simulink model "BE_EGAL_04"  (R2024b)
settings: Solver=ode45  StartTime=0.0  StopTime=1000  RelTol=1e-3  EnableMultiTasking=on
values from neighbouring files (symbols this model uses):
  Constellation = exp(1i*pi*(1+2*kc)/4)    [init_ISI.m]
undefined symbols (not defined in the file or in its folder): dfilt, Kegal, NCoeffs, Tfinal
libraries: dspobslib x3, commdigbbndam3 x3, commsink2 x2, commchan3 x1, dspstat3 x1, dspswit3 x1, commrandsrc3 x1
settings Model: Creator=Epsilon_2  LastModifiedBy=paulj
settings SolverCC: AlgebraicLoopSolver=TrustRegion
settings DataIOCC: LimitDataPoints=on  SaveFormat=Array  SignalLoggingSaveFormat=ModelDataLogs  SaveOutput=off  SaveTime=off  ReturnWorkspaceOutputs=off  SignalLoggingName=sigsOut
settings OptimizationCC: ExpressionDepthLimit=2147483647  InitFltsAndDblsToZero=on  LifeSpan=inf
settings DebuggingCC: SaveWithParameterizedLinksMsg=none  UnderspecifiedInitializationDetection=Classic  MergeDetectMultiDrivingBlocksExec=none  SignalResolutionControl=TryResolveAllWithWarning  MultiTaskDSMMsg=warning  MultiTaskCondExecSysMsg=none  FcnCallInpInsideContextMsg=warning  UnconnectedInputMsg=warning  UnconnectedOutputMsg=warning  UnconnectedLineMsg=warning  StateNameClashWarn=warning  SFUnexpectedBacktrackingDiag=warning  SFNoUnconditionalDefaultTransitionDiag=warning  SFExecutionAtInitializationDiag=none  ArithmeticOperatorsInVariantConditions=warning
settings HardwareCC: ProdBitPerPointer=32  ProdBitPerSizeT=32  ProdBitPerPtrDiffT=32  ProdLargestAtomicFloat=None  ProdIntDivRoundTo=Undefined  ProdEndianess=Unspecified  ProdWordSize=32  ProdHWDeviceType=32-bit Generic  TargetUnknown=on
settings ModelReferenceCC: PropagateSignalLabelsOutOfModel=off
settings RTWCC: GPUComputeCapability=3.5
settings CodeAppCC: StateflowObjectComments=on
settings GRTTargetCC: TargetFcnLib=ansi_tfl_tmw.mat  TargetLangStandard=C89/C90 (ANSI)  ModelReferenceCompliant=off  CombineOutputUpdateFcns=off  MatFileLogging=off  GRTInterface=on
settings ConfigComp: CovMetricSettings=dw  CovSaveCumulativeToWorkspaceVar=on  CovSaveSingleToWorkspaceVar=on

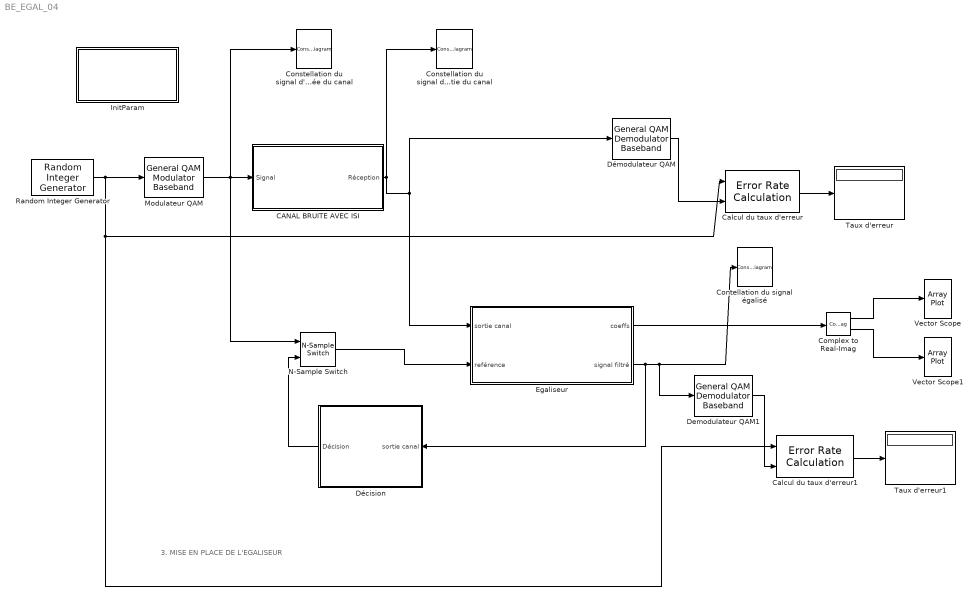
== system BE_EGAL_04 ==
  note: 3. MISE EN PLACE DE L'EGALISEUR
  CANAL BRUITE AVEC ISI : Subsystem
  Calcul du taux d'erreur : commsink2/Error Rate Calculation  N=0  st_delay=0  cp_mode=Entire frame  subframe=[]  PMode=Port  WsName=ErrorVec  RsMode2=off  stop=off  numErr=100  maxBits=1e6
  Calcul du taux d'erreur1 : commsink2/Error Rate Calculation  N=0  st_delay=0  cp_mode=Entire frame  subframe=[]  PMode=Port  WsName=ErrorVec  RsMode2=off  stop=off  numErr=100  maxBits=1e6
  Complex to Real-Imag : ComplexToRealImag
  Constellation du signal d'entrée du canal : ConstellationDiagram  Tag=ScatterPlot  WindowPosition=[382.000000,84.000000,600.000000,600.000000,]  Visible=on  ScopeFrameLocation=window  SymbolsToDisplaySource=Property  SymbolsToDisplay=1000  XLimits=[-1.47,1.47]  YLimits=[-1.38,1.38]  FigPos=[232 118 560 560]
  Constellation du signal de sortie du canal : ConstellationDiagram  Tag=ScatterPlot  WindowPosition=[463.000000,136.000000,600.000000,600.000000,]  Visible=on  ScopeFrameLocation=window  SymbolsToDisplaySource=Property  SymbolsToDisplay=1000  XLimits=[-1.47,1.47]  YLimits=[-1.38,1.38]  FigPos=[232 118 560 560]
  Contellation du signal égalisé : ConstellationDiagram  Tag=ScatterPlot  WindowPosition=[1161.000000,252.000000,600.000000,600.000000,]  Visible=on  ScopeFrameLocation=window  SymbolsToDisplaySource=Property  SymbolsToDisplay=1000  XLimits=[-1.47,1.47]  YLimits=[-1.38,1.38]  FigPos=[232 118 560 560]
  Demodulateur QAM1 : commdigbbndam3/General QAM Demodulator Baseband  SigCon=Constellation  OutType=Integer  DecType=Hard decision  VarSource=Dialog  Variance=1  outDtypeBit=Inherit via internal rule  outDtype=double  roundingMode=Floor  overflowMode=Wrap  OvFlMode=off  OvFlModeLastStrValue=off  sigConstWordLen=16  sigConstDataTypeStr=Inherit: Same word length as input  sigConstLastDataTypeStr=Inherit: Same word length as input  accum1WordLen=32  accum1FracLen=30  prodInWordLen=32  prodInFracLen=30  prodInDataTypeStr=Inherit: Same as accumulator 1  prodInLastDataTypeStr=Inherit: Same as accumulator 1  prodOutWordLen=32  prodOutFracLen=30  accum2WordLen=32  accum2FracLen=30  accum3WordLen=32  accum3FracLen=30  nsiWordLen=32  nsiFracLen=30  nsiDataTypeStr=Inherit: Same as accumulator 3  nsiLastDataTypeStr=Inherit: Same as accumulator 3  invn0WordLen=16  invn0FracLen=8  invn0DataTypeStr=Inherit: Same word length as input  invn0LastDataTypeStr=Inherit: Same word length as input  outputWordLen=32  outputFracLen=30
  Décision : Subsystem
  "Démodulateur QAM " : commdigbbndam3/General QAM Demodulator Baseband  SigCon=Constellation  OutType=Integer  DecType=Hard decision  VarSource=Dialog  Variance=1  outDtypeBit=Inherit via internal rule  outDtype=double  roundingMode=Floor  overflowMode=Wrap  OvFlMode=off  OvFlModeLastStrValue=off  sigConstWordLen=16  sigConstDataTypeStr=Inherit: Same word length as input  sigConstLastDataTypeStr=Inherit: Same word length as input  accum1WordLen=32  accum1FracLen=30  prodInWordLen=32  prodInFracLen=30  prodInDataTypeStr=Inherit: Same as accumulator 1  prodInLastDataTypeStr=Inherit: Same as accumulator 1  prodOutWordLen=32  prodOutFracLen=30  accum2WordLen=32  accum2FracLen=30  accum3WordLen=32  accum3FracLen=30  nsiWordLen=32  nsiFracLen=30  nsiDataTypeStr=Inherit: Same as accumulator 3  nsiLastDataTypeStr=Inherit: Same as accumulator 3  invn0WordLen=16  invn0FracLen=8  invn0DataTypeStr=Inherit: Same word length as input  invn0LastDataTypeStr=Inherit: Same word length as input  outputWordLen=32  outputFracLen=30
  Egaliseur : Subsystem
  InitParam : Subsystem  mask{Tech=1, Tfinal=1000, Mconst=4, NumCanal=[1 0.75 0.56 0.42 0.32 0.24 0.18], SNRcanal=100, NCoeffs=9, Kegal=0.04}
      mask prompts: Tech "Période de symbole"; Tfinal "Temps de simulation"; Mconst "Taille de la constellation de la modulation QAM : M (2^k)"; NumCanal "Modele RIF du canal"; SNRcanal "SNR du canal (en dB)"; NCoeffs "Nb de coefficients de l'égalisateur"; Kegal "Gain de l'égalisateur"
      mask help: Use the following mask to select the different parameters for the simulation.
      mask init:
      | eStr = init_ISI(gcb);
      mask Display: disp('Initialisation')
  "Modulateur QAM " : commdigbbndam3/General QAM Modulator Baseband  SigCon=Constellation  outDtype=double  outWordLen=16  outUDDataType=sfix(16)  outFracLenMode=Best precision  outFracLen=15  outDataTypeStr=double  outLastDataTypeStr=double
  N-Sample Switch : dspswit3/N-Sample Switch  N=Tfinal/10  reset=off  TriggerType=Rising edge  Ts=-1
  Random Integer Generator : commrandsrc3/Random Integer Generator  SetSize=4  SeedSource=Auto  Seed=0  SampleTime=1  SamplesPerFrame=1  OutputDataType=double  SimulateUsing=Interpreted execution
  Taux d'erreur : Display
  Taux d'erreur1 : Display
  Vector Scope : ArrayPlot  WindowPosition=[108.000000,461.000000,531.000000,480.000000,]  Visible=on  ScopeFrameLocation=window  PlotType=Line  XLabel=Time  YLimits=[-0.9705 1.2189]
  Vector Scope1 : ArrayPlot  WindowPosition=[688.000000,480.000000,484.000000,479.000000,]  Visible=on  ScopeFrameLocation=window  PlotType=Line  XLabel=Time  YLimits=[-0.0041 0.004]
  wires:
  CANAL BRUITE AVEC ISI/1(Réception) -> Constellation du signal de sortie du canal/1, "Démodulateur QAM "/1, Egaliseur/1(sortie canal)
  Random Integer Generator/1 -> "Modulateur QAM "/1, Calcul du taux d'erreur/1, Calcul du taux d'erreur1/1
  "Modulateur QAM "/1 -> N-Sample Switch/1, CANAL BRUITE AVEC ISI/1(Signal), Constellation du signal d'entrée du canal/1
  Calcul du taux d'erreur/1 -> Taux d'erreur/1
  "Démodulateur QAM "/1 -> Calcul du taux d'erreur/2
  Egaliseur/1(coeffs) -> Complex to Real-Imag/1
  Complex to Real-Imag/1 -> Vector Scope/1
  Complex to Real-Imag/2 -> Vector Scope1/1
  Calcul du taux d'erreur1/1 -> Taux d'erreur1/1
  Demodulateur QAM1/1 -> Calcul du taux d'erreur1/2
  Egaliseur/2(signal filtré) -> Décision/1(sortie canal), Demodulateur QAM1/1, Contellation du signal égalisé/1
  Décision/1(Décision) -> N-Sample Switch/2
  N-Sample Switch/1 -> Egaliseur/2(reférence)

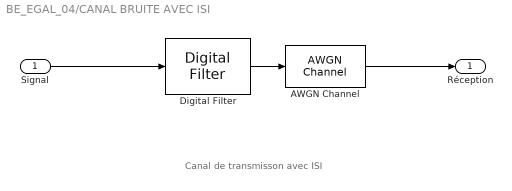
== system BE_EGAL_04/CANAL BRUITE AVEC ISI ==
  note: Canal de transmisson avec ISI
  Signal : Inport
  AWGN Channel : commchan3/AWGN Channel  LegacyMode=on  NoiseMethod="Signal to noise ratio  (SNR)"  noiseMode="Signal to noise ratio  (SNR)"  EbNo=10  EsNo=10  SNR=SNRcanal  BitsPerSymbol=1  SignalPower=1  SamplesPerSymbol=1  SymbolPeriod=1  VarianceSource=Parameter  Variance=1  RandomStream=Global stream  Seed=67  SimulateUsing=Code generation
  Digital Filter : dspobslib/Digital Filter  TypePopup=FIR (all zeros)  IIRFiltStruct=Direct form II transposed  AllPoleFiltStruct=Direct form  FIRFiltStruct=Direct form  CoeffSource=Specify via dialog  NumCoeffs=NumCanal  DenCoeffs=[1 0.1]  BiQuadCoeffs=[1 0.3 0.4 1 0.1 0.2]  LatticeCoeffs=[0.2 0.4]  denIgnore=on  FiltPerSampPopup=One filter per sample  IC=0  ICnum=0  ICden=0  roundingMode=Floor  overflowMode=off  ScaleValues=1  scaleValueFracLength=14  stageInFracLength=15  stageOutFracLength=15  FilterSource=Specify via dialog  dfiltObjectName=dfilt.dffir([1 2 1])  InputProcessing=Columns as channels (frame based)
  Réception : Outport
  wires:
  Digital Filter/1 -> AWGN Channel/1
  AWGN Channel/1 -> Réception/1
  Signal/1 -> Digital Filter/1

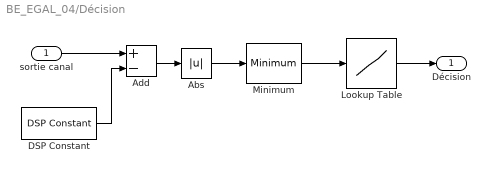
== system BE_EGAL_04/Décision ==
  sortie canal : Inport
  Abs : Abs  SaturateOnIntegerOverflow=off
  Add : Sum  Inputs=+-
  DSP Constant : dspobslib/DSP Constant  Value=Constellation  SampleMode=Discrete  discreteOutput=Sample-based (interpret vectors as 1-D)  continuousOutput=Sample-based  sampTime=inf  framePeriod=2  dataType=Inherit from 'Constant value'  isSigned=on  wordLen=16  udDataType=sfix(16)  fracBitsMode=Best precision  numFracBits=15  InterpretAs1D=-inf  Ts=-inf  FramebasedOutput=-inf
  Lookup Table : Lookup  InputValues=[1:4]  Table=Constellation  LookUpMeth=Use Input Nearest  SaturateOnIntegerOverflow=off
  Minimum : dspstat3/Minimum  operation=minimum  fcn=Index  indexBase=One  operateOver=Each column  Dimension=1  InputProcessing=Columns as channels (frame based)  reset=None  roiEnable=off  roiType=Rectangles  roiPortion=Entire ROI  roiOutput=Individual statistics for each ROI  roiFlag=off  roundingMode=Floor  overflowMode=off
  Décision : Outport
  wires:
  Minimum/1 -> Lookup Table/1
  Lookup Table/1 -> Décision/1
  Abs/1 -> Minimum/1
  Add/1 -> Abs/1
  DSP Constant/1 -> Add/2
  sortie canal/1 -> Add/1

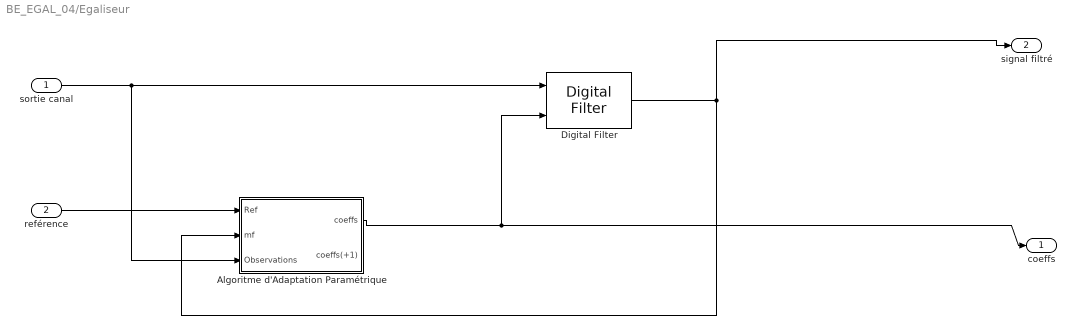
== system BE_EGAL_04/Egaliseur ==
  sortie canal : Inport
  reférence : Inport  Port=2
  Algoritme d'Adaptation Paramétrique : Subsystem
  Digital Filter : dspobslib/Digital Filter  TypePopup=FIR (all zeros)  IIRFiltStruct=Direct form II transposed  AllPoleFiltStruct=Direct form  FIRFiltStruct=Direct form  CoeffSource=Input port(s)  NumCoeffs=1  DenCoeffs=[1 0.1]  BiQuadCoeffs=[1 0.3 0.4 1 0.1 0.2]  LatticeCoeffs=[0.2 0.4]  denIgnore=on  FiltPerSampPopup=One filter per sample  IC=0  ICnum=0  ICden=0  roundingMode=Floor  overflowMode=off  ScaleValues=1  scaleValueFracLength=14  stageInFracLength=15  stageOutFracLength=15  FilterSource=Input port(s)  dfiltObjectName=dfilt.dffir([1 2 1])  InputProcessing=Columns as channels (frame based)
  coeffs : Outport
  signal filtré : Outport  Port=2
  wires:
  sortie canal/1 -> Digital Filter/1, Algoritme d'Adaptation Paramétrique/3(Observations)
  Algoritme d'Adaptation Paramétrique/1(coeffs) -> Digital Filter/2, coeffs/1
  reférence/1 -> Algoritme d'Adaptation Paramétrique/1(Ref)
  Digital Filter/1 -> signal filtré/1, Algoritme d'Adaptation Paramétrique/2(mf)

== system BE_EGAL_04/InitParam ==

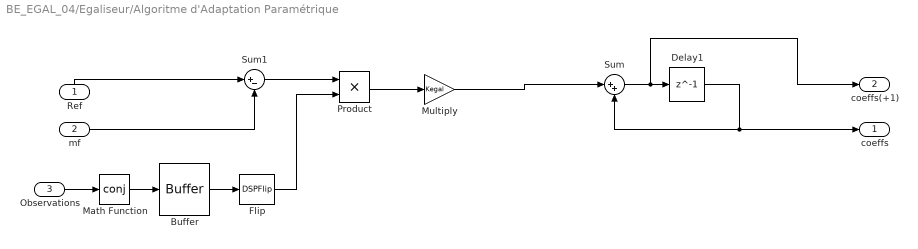
== system BE_EGAL_04/Egaliseur/Algoritme d'Adaptation Paramétrique ==
  Ref : Inport
  mf : Inport  Port=2
  Observations : Inport  Port=3
  Buffer : Buffer  N=NCoeffs  V=NCoeffs-1  OutputFrames=off
  Delay1 : Delay  DelayLength=1
  Flip : DSPFlip
  Math Function : Math  Operator=conj
  Multiply : Gain  Gain=Kegal
  Product : Product
  Sum : Sum  Inputs=|++
  Sum1 : Sum  Inputs=|+-
  coeffs : Outport
  coeffs(+1) : Outport  Port=2
  wires:
  Ref/1 -> Sum1/1
  mf/1 -> Sum1/2
  Sum1/1 -> Product/1
  Product/1 -> Multiply/1
  Multiply/1 -> Sum/1
  Sum/1 -> coeffs(+1)/1, Delay1/1
  Observations/1 -> Math Function/1
  Buffer/1 -> Flip/1
  Flip/1 -> Product/2
  Delay1/1 -> Sum/2, coeffs/1
  Math Function/1 -> Buffer/1
